simulink model "insModel"  (R2019a)
settings: Solver=FixedStepDiscrete  StartTime=0.0  StopTime=10.0  FixedStep=Ts  RelTol=1e-3
values from neighbouring files (symbols this model uses):
  acc_var = 0.01    [IMU_init.m]
  accel_fullscale = 4*g    (= 39.24)    [IMU_init.m]
  ba = [bax; bay; baz]    [IMU_init.m]
  bar_var = 10    [BARO_init.m]
  baro_fullscale = 4800e3    (= 4800000)    [BARO_init.m]
  bb = 0    [BARO_init.m]
  bg = [bgx; bgy; bgz]    [IMU_init.m]
  bgps = [2;2;0.5]    [GPS_init.m]
  bm = [bmx; bmy; bmz]    [IMU_init.m]
  gavity_ned = [0; 0; g]    [IMU_init.m]
  gps_var = [0.001;0.001;0.001]    [GPS_init.m]
  gyr_var = 0.01    [IMU_init.m]
  gyro_fullscale = 500*pi/180    (= 8.72664625997)    [IMU_init.m]
  Ma = eye(3)    [IMU_init.m]
  mag_fullscale = 4800e3    (= 4800000)    [IMU_init.m]
  mag_ned = [22854.5;971.8;41394.7]    [IMU_init.m]
  mag_var = 0.01    [IMU_init.m]
  Mg = [1     Mgxy     Mgxz ... (first row only)    [IMU_init.m]
  Mm = [1     Mmxy     Mmxz ... (first row only)    [IMU_init.m]
  realSensorBaro = 1    [BARO_init.m]
  realSensorGPS = 1    [GPS_init.m]
  realSensorIMU = 1    [IMU_init.m]
  Sa = eye(3)    [IMU_init.m]
  Sb = 1    [BARO_init.m]
  seed_ax = abs(randi(1e4))    [IMU_init.m]
  seed_ay = abs(randi(1e4))    [IMU_init.m]
  seed_az = abs(randi(1e4))    [IMU_init.m]
  seed_b = abs(randi(1e4))    [BARO_init.m]
  seed_gpsx = abs(randi(1e4))    [GPS_init.m]
  seed_gpsy = abs(randi(1e4))    [GPS_init.m]
  seed_gpsz = abs(randi(1e4))    [GPS_init.m]
  seed_gx = abs(randi(1e4))    [IMU_init.m]
  seed_gy = abs(randi(1e4))    [IMU_init.m]
  seed_gz = abs(randi(1e4))    [IMU_init.m]
  seed_mx = abs(randi(1e4))    [IMU_init.m]
  seed_my = abs(randi(1e4))    [IMU_init.m]
  seed_mz = abs(randi(1e4))    [IMU_init.m]
  Sg = diag([Sgx;Sgy; Sgz])    [IMU_init.m]
  Sm = diag([Smx;Smy; Smz])    [IMU_init.m]
  Ts = 4e-3    (= 0.004)    [IMU_init.m]
settings Model: Creator=matte  LastModifiedBy=david
settings DataIOCC: ReturnWorkspaceOutputs=off
settings DebuggingCC: ArithmeticOperatorsInVariantConditions=warning
settings SFSimCC: SimUseLocalCustomCode=off
settings RTWCC: RTWUseLocalCustomCode=off
settings CodeAppCC: StateflowObjectComments=on

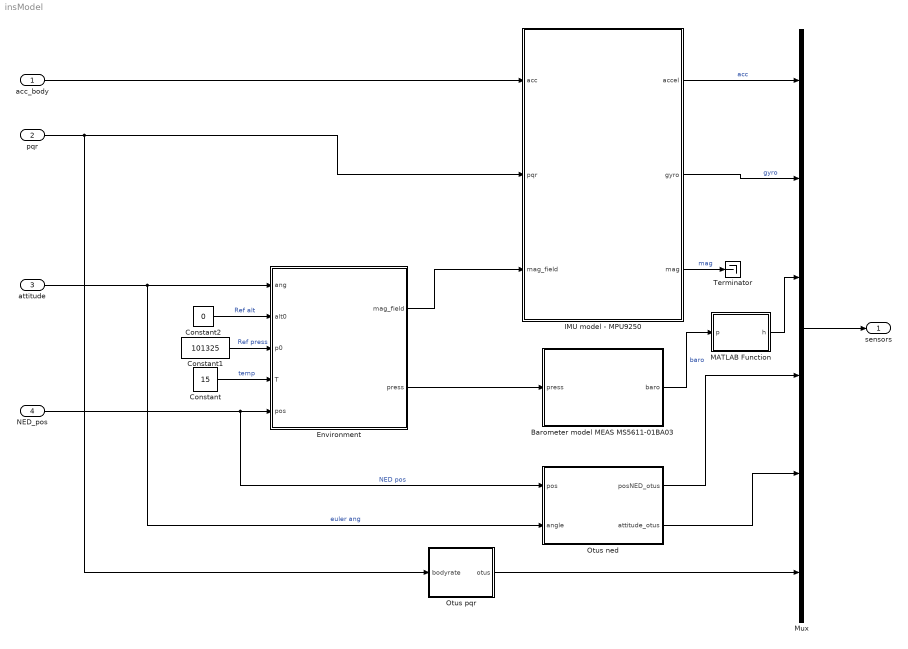
== system insModel ==
  acc_body : Inport  PortDimensions=3
  pqr : Inport  Port=2  PortDimensions=3
  attitude : Inport  Port=3  PortDimensions=3
  NED_pos : Inport  Port=4  PortDimensions=3
  Barometer model MEAS MS5611-01BA03 : Subsystem
      mask Display: %image('img\baroMEAS.jpg');
  Constant : Constant  Value=15
  Constant1 : Constant  Value=101325
  Constant2 : Constant  Value=0
  Environment : Subsystem
  IMU model - MPU9250 : Subsystem
      mask Display: %image('img\mpu9250.jpg');
  MATLAB Function : MATLAB Function  TreatAsAtomicUnit=on
  Mux : Mux  Inputs=6
  Otus ned : Subsystem
      mask Display: %image('img\ublox.jpg');
  Otus pqr : Subsystem
  Terminator : Terminator
  sensors : Outport
  wires:
  Environment/1(mag_field) -> IMU model - MPU9250/3(mag_field)
  IMU model - MPU9250/1(accel) -> Mux/1  "acc"
  IMU model - MPU9250/2(gyro) -> Mux/2  "gyro"
  IMU model - MPU9250/3(mag) -> Terminator/1  "mag"
  Mux/1 -> sensors/1
  Constant/1 -> Environment/4(T)  "temp"
  Constant1/1 -> Environment/3(p0)  "Ref press"
  Constant2/1 -> Environment/2(alt0)  "Ref alt"
  NED_pos/1 -> Otus ned/1(pos), Environment/5(pos)  "NED pos"
  attitude/1 -> Otus ned/2(angle), Environment/1(ang)  "euler ang"
  Environment/2(press) -> Barometer model MEAS MS5611-01BA03/1(press)
  Barometer model MEAS MS5611-01BA03/1(baro) -> MATLAB Function/1(p)  "baro"
  Otus ned/1(posNED_otus) -> Mux/4
  acc_body/1 -> IMU model - MPU9250/1(acc)
  Otus pqr/1(otus) -> Mux/6
  pqr/1 -> Otus pqr/1(bodyrate), IMU model - MPU9250/2(pqr)
  MATLAB Function/1(h) -> Mux/3
  Otus ned/2(attitude_otus) -> Mux/5

== system insModel/Barometer model MEAS MS5611-01BA03 ==
  press : Inport
  Barometer : Subsystem
  Rate Transition2 : RateTransition
  baro : Outport
  wires:
  press/1 -> Barometer/1(press)
  Rate Transition2/1 -> baro/1
  Barometer/1(baro) -> Rate Transition2/1

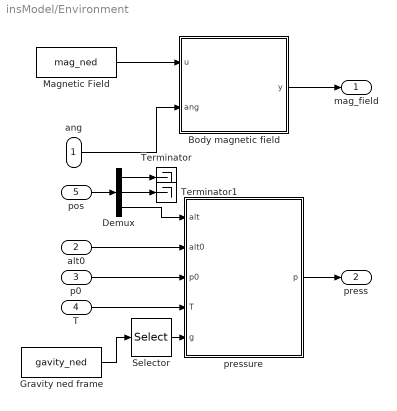
== system insModel/Environment ==
  ang : Inport
  alt0 : Inport  Port=2
  p0 : Inport  Port=3
  T : Inport  Port=4
  pos : Inport  Port=5
  Body magnetic field : MATLAB Function  TreatAsAtomicUnit=on
  Demux : Demux  Outputs=3
  Gravity ned frame : Constant  Value=gavity_ned
  Magnetic Field : Constant  Value=mag_ned
  Selector : Selector  InputPortWidth=3  IndexOptions=Index vector (dialog)  Indices=[3]  OutputSizes=1
  Terminator : Terminator
  Terminator1 : Terminator
  pressure : MATLAB Function  TreatAsAtomicUnit=on
  mag_field : Outport
  press : Outport  Port=2
  wires:
  Body magnetic field/1(y) -> mag_field/1
  pressure/1(p) -> press/1
  ang/1 -> Body magnetic field/2(ang)
  Magnetic Field/1 -> Body magnetic field/1(u)
  pos/1 -> Demux/1
  Demux/3 -> pressure/1(alt)
  Demux/1 -> Terminator/1
  Demux/2 -> Terminator1/1
  Gravity ned frame/1 -> Selector/1
  alt0/1 -> pressure/2(alt0)
  p0/1 -> pressure/3(p0)
  T/1 -> pressure/4(T)
  Selector/1 -> pressure/5(g)

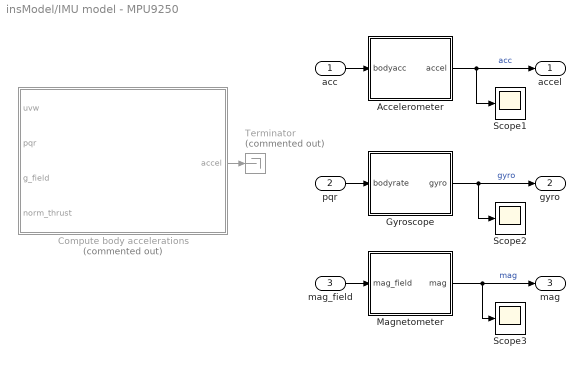
== system insModel/IMU model - MPU9250 ==
  acc : Inport
  pqr : Inport  Port=2
  mag_field : Inport  Port=3
  Accelerometer : Subsystem
  "Compute body accelerations " : MATLAB Function  Commented=on  TreatAsAtomicUnit=on
  Gyroscope : Subsystem
  Magnetometer : Subsystem
  Scope1 : Scope
  Scope2 : Scope
  Scope3 : Scope
  Terminator : Terminator  Commented=on
  accel : Outport
  gyro : Outport  Port=2
  mag : Outport  Port=3
  wires:
  acc/1 -> Accelerometer/1(bodyacc)
  pqr/1 -> Gyroscope/1(bodyrate)
  mag_field/1 -> Magnetometer/1(mag_field)
  Accelerometer/1(accel) -> accel/1, Scope1/1  "acc"
  Gyroscope/1(gyro) -> Scope2/1, gyro/1  "gyro"
  Magnetometer/1(mag) -> Scope3/1, mag/1  "mag"
  "Compute body accelerations "/1(accel) -> Terminator/1

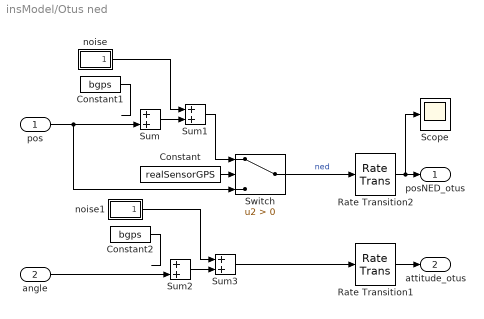
== system insModel/Otus ned ==
  pos : Inport
  angle : Inport  Port=2
  Constant : Constant  Value=realSensorGPS
  Constant1 : Constant  Value=bgps
  Constant2 : Constant  Value=bgps
  Rate Transition1 : RateTransition
  Rate Transition2 : RateTransition
  Scope : Scope
  Sum{,1..3} (4 alike) : Sum
  Switch : Switch  Criteria=u2 > Threshold
  noise : Subsystem
  noise1 : Subsystem
  posNED_otus : Outport
  attitude_otus : Outport  Port=2
  wires:
  Rate Transition1/1 -> attitude_otus/1
  noise/1(noise) -> Sum1/1
  Sum3/1 -> Rate Transition1/1
  Sum2/1 -> Sum3/2
  pos/1 -> Sum/2, Switch/3
  Constant2/1 -> ?
  Rate Transition2/1 -> Scope/1, posNED_otus/1
  Sum1/1 -> Switch/1
  Constant/1 -> Switch/2
  Sum/1 -> Sum1/2
  Constant1/1 -> ?
  angle/1 -> Sum2/2
  noise1/1(noise) -> Sum3/1
  Switch/1 -> Rate Transition2/1  "ned"

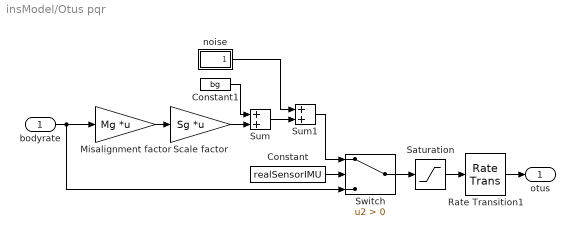
== system insModel/Otus pqr ==
  bodyrate : Inport
  Constant : Constant  Value=realSensorIMU
  Constant1 : Constant  Value=bg
  Misalignment factor : Gain  Gain=Mg  Multiplication=Matrix(K*u)
  Rate Transition1 : RateTransition
  Saturation : Saturate  UpperLimit=gyro_fullscale  LowerLimit=-accel_fullscale
  Scale factor : Gain  Gain=Sg  Multiplication=Matrix(K*u)
  Sum : Sum
  Sum1 : Sum
  Switch : Switch  Criteria=u2 > Threshold
  noise : Subsystem
  otus : Outport
  wires:
  Switch/1 -> Saturation/1
  Constant/1 -> Switch/2
  Sum/1 -> Sum1/2
  Scale factor/1 -> Sum/2
  Constant1/1 -> Sum/1
  noise/1(noise) -> Sum1/1
  Sum1/1 -> Switch/1
  bodyrate/1 -> Misalignment factor/1, Switch/3
  Misalignment factor/1 -> Scale factor/1
  Saturation/1 -> Rate Transition1/1
  Rate Transition1/1 -> otus/1

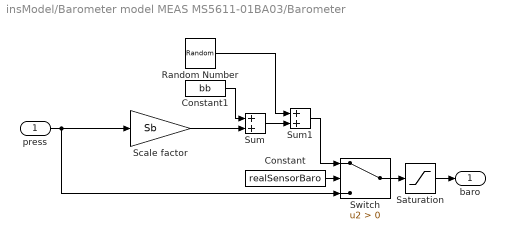
== system insModel/Barometer model MEAS MS5611-01BA03/Barometer ==
  press : Inport
  Constant : Constant  Value=realSensorBaro
  Constant1 : Constant  Value=bb
  Random Number : RandomNumber  Variance=bar_var  Seed=seed_b  SampleTime=Ts
  Saturation : Saturate  UpperLimit=baro_fullscale  LowerLimit=-accel_fullscale
  Scale factor : Gain  Gain=Sb
  Sum : Sum
  Sum1 : Sum
  Switch : Switch  Criteria=u2 > Threshold
  baro : Outport
  wires:
  press/1 -> Switch/3, Scale factor/1
  Sum1/1 -> Switch/1
  Random Number/1 -> Sum1/1
  Constant1/1 -> Sum/1
  Scale factor/1 -> Sum/2
  Sum/1 -> Sum1/2
  Constant/1 -> Switch/2
  Switch/1 -> Saturation/1
  Saturation/1 -> baro/1

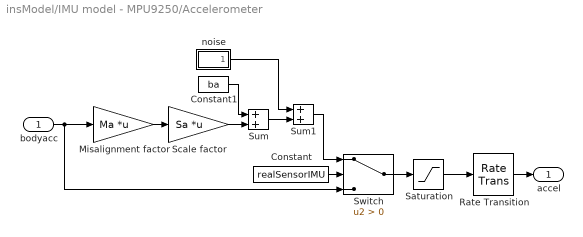
== system insModel/IMU model - MPU9250/Accelerometer ==
  bodyacc : Inport
  Constant : Constant  Value=realSensorIMU
  Constant1 : Constant  Value=ba
  Misalignment factor : Gain  Gain=Ma  Multiplication=Matrix(K*u)
  Rate Transition : RateTransition
  Saturation : Saturate  UpperLimit=accel_fullscale  LowerLimit=-accel_fullscale
  Scale factor : Gain  Gain=Sa  Multiplication=Matrix(K*u)
  Sum : Sum
  Sum1 : Sum
  Switch : Switch  Criteria=u2 > Threshold
  noise : Subsystem
  accel : Outport
  wires:
  Misalignment factor/1 -> Scale factor/1
  bodyacc/1 -> Switch/3, Misalignment factor/1
  Sum1/1 -> Switch/1
  Constant1/1 -> Sum/1
  Scale factor/1 -> Sum/2
  Sum/1 -> Sum1/2
  Constant/1 -> Switch/2
  Switch/1 -> Saturation/1
  noise/1(noise) -> Sum1/1
  Saturation/1 -> Rate Transition/1
  Rate Transition/1 -> accel/1

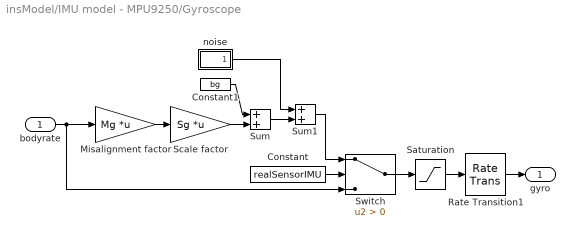
== system insModel/IMU model - MPU9250/Gyroscope ==
  bodyrate : Inport
  Constant : Constant  Value=realSensorIMU
  Constant1 : Constant  Value=bg
  Misalignment factor : Gain  Gain=Mg  Multiplication=Matrix(K*u)
  Rate Transition1 : RateTransition
  Saturation : Saturate  UpperLimit=gyro_fullscale  LowerLimit=-accel_fullscale
  Scale factor : Gain  Gain=Sg  Multiplication=Matrix(K*u)
  Sum : Sum
  Sum1 : Sum
  Switch : Switch  Criteria=u2 > Threshold
  noise : Subsystem
  gyro : Outport
  wires:
  Switch/1 -> Saturation/1
  Constant/1 -> Switch/2
  Sum/1 -> Sum1/2
  Scale factor/1 -> Sum/2
  Constant1/1 -> Sum/1
  noise/1(noise) -> Sum1/1
  Sum1/1 -> Switch/1
  bodyrate/1 -> Misalignment factor/1, Switch/3
  Misalignment factor/1 -> Scale factor/1
  Saturation/1 -> Rate Transition1/1
  Rate Transition1/1 -> gyro/1

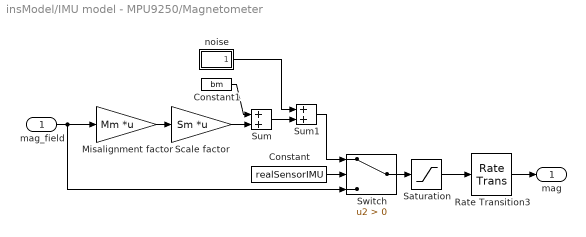
== system insModel/IMU model - MPU9250/Magnetometer ==
  mag_field : Inport
  Constant : Constant  Value=realSensorIMU
  Constant1 : Constant  Value=bm
  Misalignment factor : Gain  Gain=Mm  Multiplication=Matrix(K*u)
  Rate Transition3 : RateTransition
  Saturation : Saturate  UpperLimit=mag_fullscale  LowerLimit=-mag_fullscale
  Scale factor : Gain  Gain=Sm  Multiplication=Matrix(K*u)
  Sum : Sum
  Sum1 : Sum
  Switch : Switch  Criteria=u2 > Threshold
  noise : Subsystem
  mag : Outport
  wires:
  Switch/1 -> Saturation/1
  Constant/1 -> Switch/2
  Sum/1 -> Sum1/2
  Scale factor/1 -> Sum/2
  Constant1/1 -> Sum/1
  noise/1(noise) -> Sum1/1
  Sum1/1 -> Switch/1
  mag_field/1 -> Misalignment factor/1, Switch/3
  Misalignment factor/1 -> Scale factor/1
  Saturation/1 -> Rate Transition3/1
  Rate Transition3/1 -> mag/1

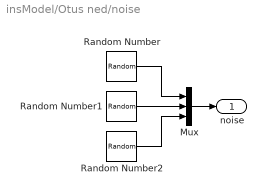
== system insModel/Otus ned/noise ==
  Mux : Mux  Inputs=3
  Random Number : RandomNumber  Variance=gps_var(1)  Seed=seed_gpsx  SampleTime=Ts
  Random Number1 : RandomNumber  Variance=gps_var(2)  Seed=seed_gpsy  SampleTime=Ts
  Random Number2 : RandomNumber  Variance=gps_var(3)  Seed=seed_gpsz  SampleTime=Ts
  noise : Outport
  wires:
  Random Number1/1 -> Mux/2
  Random Number/1 -> Mux/1
  Mux/1 -> noise/1
  Random Number2/1 -> Mux/3

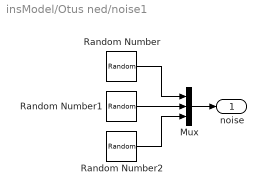
== system insModel/Otus ned/noise1 ==
  Mux : Mux  Inputs=3
  Random Number : RandomNumber  Variance=gps_var(1)  Seed=seed_gpsx  SampleTime=Ts
  Random Number1 : RandomNumber  Variance=gps_var(2)  Seed=seed_gpsy  SampleTime=Ts
  Random Number2 : RandomNumber  Variance=gps_var(3)  Seed=seed_gpsz  SampleTime=Ts
  noise : Outport
  wires:
  Random Number1/1 -> Mux/2
  Random Number/1 -> Mux/1
  Mux/1 -> noise/1
  Random Number2/1 -> Mux/3

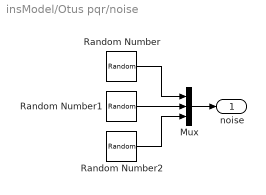
== system insModel/Otus pqr/noise ==
  Mux : Mux  Inputs=3
  Random Number : RandomNumber  Variance=gyr_var  Seed=seed_gx  SampleTime=Ts
  Random Number1 : RandomNumber  Variance=gyr_var  Seed=seed_gy  SampleTime=Ts
  Random Number2 : RandomNumber  Variance=gyr_var  Seed=seed_gz  SampleTime=Ts
  noise : Outport
  wires:
  Random Number1/1 -> Mux/2
  Random Number/1 -> Mux/1
  Mux/1 -> noise/1
  Random Number2/1 -> Mux/3

== system insModel/IMU model - MPU9250/Accelerometer/noise ==
  Mux : Mux  Inputs=3
  Random Number : RandomNumber  Variance=acc_var  Seed=seed_ax  SampleTime=Ts
  Random Number1 : RandomNumber  Variance=acc_var  Seed=seed_ay  SampleTime=Ts
  Random Number2 : RandomNumber  Variance=acc_var  Seed=seed_az  SampleTime=Ts
  noise : Outport
  wires:
  Random Number1/1 -> Mux/2
  Random Number/1 -> Mux/1
  Mux/1 -> noise/1
  Random Number2/1 -> Mux/3

== system insModel/IMU model - MPU9250/Gyroscope/noise ==
  Mux : Mux  Inputs=3
  Random Number : RandomNumber  Variance=gyr_var  Seed=seed_gx  SampleTime=Ts
  Random Number1 : RandomNumber  Variance=gyr_var  Seed=seed_gy  SampleTime=Ts
  Random Number2 : RandomNumber  Variance=gyr_var  Seed=seed_gz  SampleTime=Ts
  noise : Outport
  wires:
  Random Number1/1 -> Mux/2
  Random Number/1 -> Mux/1
  Mux/1 -> noise/1
  Random Number2/1 -> Mux/3

== system insModel/IMU model - MPU9250/Magnetometer/noise ==
  Mux : Mux  Inputs=3
  Random Number : RandomNumber  Variance=mag_var  Seed=seed_mx  SampleTime=Ts
  Random Number1 : RandomNumber  Variance=mag_var  Seed=seed_my  SampleTime=Ts
  Random Number2 : RandomNumber  Variance=mag_var  Seed=seed_mz  SampleTime=Ts
  noise : Outport
  wires:
  Random Number1/1 -> Mux/2
  Random Number/1 -> Mux/1
  Mux/1 -> noise/1
  Random Number2/1 -> Mux/3

== matlab function insModel/MATLAB Function ==
  data: p input; h output
function h = press2alt(p)

p0 = 101325;
R_air = 286.9;
T0 = 288.15;

h = -R_air*T0/9.81*log(p/p0);
end

== matlab function insModel/Environment/Body magnetic field ==
  data: u input; y output; ang input
function y = ned2body(u,ang)
%--------------------------------------------------------------------------
% Author: Matteo Scanavino (matteo.scanavino@polito.it)
% Affiliation: Politecnico di Torino - Department of Mechanical and
% Aerospace Engineering (DIMEAS)
% Year: 2019
% -------------------------------------------------------------------------
% 
% This function converts the u vector from the ned frame to body frame
% given the orientation of the body in Euler angles
% 
% Input:    u       ->  vector to be rotated
%           ang     ->  Euler agnle orientation
% Output:   y       ->  converted vector
%
%--------------------------------------------------------------------------

% Euler angles
phi     =   ang(1);                                                         % Roll  [rad]  
theta   =   ang(2);                                                         % Pith  [rad] 
psi     =   ang(3);                                                         % Yaw   [rad]

% Rotation matrix (form ned to body)
R       =   [cos(theta)*cos(psi)                               ...
             cos(theta)*sin(psi)                               ...       
             -sin(theta);                                      ...
             -cos(phi)*sin(psi)+sin(phi)*sin(theta)*cos(psi)   ...
             cos(phi)*cos(psi)+sin(phi)*sin(theta)*sin(psi)    ...
             sin(phi)*cos(theta);                              ...
             sin(phi)*sin(psi)+cos(phi)*sin(theta)*cos(psi)    ...
             -sin(phi)*cos(psi)+cos(phi)*sin(theta)*sin(psi)   ...
             cos(phi)*cos(theta)];
         
% Rotation 
y = R*u;

end

== matlab function insModel/Environment/pressure ==
  data: alt input; p output; alt0 input; p0 input; T input; g input
function p = pressure(alt,alt0,p0,T,g)
%--------------------------------------------------------------------------
% Author: Matteo Scanavino (matteo.scanavino@polito.it)
% Affiliation: Politecnico di Torino - Department of Mechanical and
% Aerospace Engineering (DIMEAS)
% Year: 2019
% -------------------------------------------------------------------------
% 
% This function computes ambient pressure given the altitude and
% temperature
% 
% Input:    alt     ->  altitude                    [m]
%           alt0    ->  reference altitude          [m]
%           p0      ->  pressure at reference alt   [Pa]
%           T       ->  temperature                 [°C]
%           g       ->  gravity                     [m/s^2]
% Output:   p       ->  pressure                    [Pa]
%
%--------------------------------------------------------------------------

% Air constant 
R       =       286.9; 

% Temperature conversion in Kelvin
T       =       T +273.15;                          % [K]

% Compute pressure
p       =       p0*exp((-g/(R*T))*(alt-alt0));      % [Pa]
 
end

== matlab function insModel/IMU model - MPU9250/Compute body accelerations  ==
  data: uvw input; accel output; pqr input; g_field input; norm_thrust input
function accel = acceleration(uvw,pqr,g_field,norm_thrust)
%--------------------------------------------------------------------------
% Author: Matteo Scanavino (matteo.scanavino@polito.it)
% Affiliation: Politecnico di Torino - Department of Mechanical and
% Aerospace Engineering (DIMEAS)
% Year: 2019
% -------------------------------------------------------------------------
% 
% This function simulates the Inertial Measurement Unit (imu)
% 
% Input:    uvw         ->  body velocity               [m/s]
%           pqr         ->  body angular rate           [rad/s]
%           g_field     ->  body gravity                [m/s^2]
%           norm_thrust ->  external forces             [m/s^2]
% Output:   accel       ->  boy acceleration            [m/s^2]
%
%--------------------------------------------------------------------------

% Body velocity 
u       =       uvw(1); 
v       =       uvw(2); 
w       =       uvw(3); 

% Body angular rate
p       =       pqr(1); 
q       =       pqr(2); 
r       =       pqr(3); 

% External forces normalized with respect to mass
fx      =       norm_thrust(1); 
fy      =       norm_thrust(2); 
fz      =       norm_thrust(3); 

% Gravitational field
gx      =       g_field(1); 
gy      =       g_field(2); 
gz      =       g_field(3);  

% Compute accelerations
udot    =       r*v - q*w - gx + fx;
vdot    =       -r*u + p*w + gy + fy; 
wdot    =       q*u - p*v + gz + fz; 
accel   =       [udot; vdot; wdot]; 

end
